simulink model "Target_Control_System"  (R2021b)
settings: Solver=FixedStepDiscrete  StartTime=0.0  StopTime=5  RelTol=1e-3
PreLoadFcn:
  | RTWConfigurationCB('preloadfcn', bdroot);
PostLoadFcn:
  | load('configuration/data_struct.mat');
  | load('configuration/fluxMaps_propMotor.mat');
  | load('configuration/parameterInit_PROP.mat');
  | load('configuration/parameterInit_PUMP.mat');
  | load('configuration/parameterInit_PITCH.mat');
  | load('configuration/parameterInit_TILT.mat');
  | %load('configuration/base_workspace_signal_definition.mat');
  | %load('resolvedatastores_to_baseworkspace_for_faster_simulation.mat');
model workspace (MAT data in the model file):
  SIMULATION_OPTIONS = Simulink.Parameter
  SIMULATION_OPTIONS.Value = 0
  SIMULATION_OPTIONS.Description = 'Set to ''0'' for normal Simulation
    | Set to ''1'' for "Flying Start" simulation'
  SIMULATION_OPTIONS.DataType = 'uint32'
  SIMULATION_OPTIONS.Complexity = 'real'
  SIMULATION_OPTIONS.Dimensions = [1 1]
  TARGET_CODE_GEN = Simulink.Parameter
  TARGET_CODE_GEN.Value = 0
  TARGET_CODE_GEN.Description = 'Set to ''0'' for Plant Model or PIL Simulation
    | Set to ''1'' for Target System Code Generation'
  TARGET_CODE_GEN.DataType = 'uint32'
  TARGET_CODE_GEN.Complexity = 'real'
  TARGET_CODE_GEN.Dimensions = [1 1]
  TCS_SAMPLE_FREQ_HZ = Simulink.Parameter
  TCS_SAMPLE_FREQ_HZ.Value = 160000
  TCS_SAMPLE_FREQ_HZ.DataType = 'double'
  TCS_SAMPLE_FREQ_HZ.Complexity = 'real'
  TCS_SAMPLE_FREQ_HZ.Dimensions = [1 1]
undefined symbols (not defined in the file): A_DQ_REF_LPF_INIT__PITCH, A_DQ_REF_LPF_INIT__PROP, A_DQ_REF_LPF_INIT__PUMP, A_DQ_REF_LPF_INIT__TILT, A_OBSERVER_CONFIDENCE_INIT__PITCH, A_OBSERVER_CONFIDENCE_INIT__PROP, A_OBSERVER_CONFIDENCE_INIT__PUMP, A_OBSERVER_CONFIDENCE_INIT__TILT, ACTUATOR_MAX_ANGLE_TRIP__PITCH, ACTUATOR_MIN_ANGLE_TRIP__PITCH, ACTUATOR_POS_SENSOR_INV_DIRECTION__PITCH, ACTUATOR_POS_SENSOR_INV_DIRECTION__TILT, ACTUATOR_POS_SENSOR_OFFSET__PITCH, ACTUATOR_POS_SENSOR_OFFSET__TILT, ADC_scaler1_baseaddr_TILT, ADC_SCALER_FLOAT_TO_FIXPOINT_EXPANSION, ANGLE_ELEC_FROM_SENSOR_OFFSET_INIT__PITCH, ANGLE_ELEC_FROM_SENSOR_OFFSET_INIT__PROP, ANGLE_ELEC_FROM_SENSOR_OFFSET_INIT__PUMP, ANGLE_ELEC_FROM_SENSOR_OFFSET_INIT__TILT, AUTO_CLEAR_FAULTS_ENABLED__PITCH, AUTO_CLEAR_FAULTS_ENABLED__PROP, AUTO_CLEAR_FAULTS_ENABLED__PUMP, AUTO_CLEAR_FAULTS_ENABLED__TILT, AUTO_CLEAR_FAULTS_WAIT_TICKS__PITCH, AUTO_CLEAR_FAULTS_WAIT_TICKS__PROP, AUTO_CLEAR_FAULTS_WAIT_TICKS__PUMP, AUTO_CLEAR_FAULTS_WAIT_TICKS__TILT, AUTO_I_ZERO_IDLE_TICKS__PITCH, AUTO_I_ZERO_IDLE_TICKS__PROP, AUTO_I_ZERO_IDLE_TICKS__PUMP, AUTO_I_ZERO_IDLE_TICKS__TILT, AUTO_I_ZERO_OFFSET_IDC_THRESHOLD__PITCH, AUTO_I_ZERO_OFFSET_IDC_THRESHOLD__PROP, AUTO_I_ZERO_OFFSET_IDC_THRESHOLD__PUMP, AUTO_I_ZERO_OFFSET_IDC_THRESHOLD__TILT, AUTO_I_ZERO_OFFSET_IPH_THRESHOLD__PITCH, AUTO_I_ZERO_OFFSET_IPH_THRESHOLD__PROP, AUTO_I_ZERO_OFFSET_IPH_THRESHOLD__PUMP, AUTO_I_ZERO_OFFSET_IPH_THRESHOLD__TILT, AUTO_SENSORLESS_SWITCHOVER_DISABLE_OMEGA, AUTO_SENSORLESS_SWITCHOVER_ENABLE_OMEGA, AUTO_SENSORLESS_SWITCHOVER_MIN_CONFIDENCE, AUXILIARY_PROTECTION_UNIT_BASEADDR__TILT, blanking_max_error_omega_INIT_PITCH, blanking_max_error_omega_INIT_TILT, blanking_max_error_position_INIT_PITCH, blanking_max_error_position_INIT_TILT, BRUTE_START_I_Q_REF_RAMP_SPEED__PITCH, BRUTE_START_I_Q_REF_RAMP_SPEED__PROP, BRUTE_START_I_Q_REF_RAMP_SPEED__PUMP, BRUTE_START_I_Q_REF_RAMP_SPEED__TILT, CONTROL_LOOP_DT_INIT__PITCH, CONTROL_LOOP_DT_INIT__PROP, CONTROL_LOOP_DT_INIT__PUMP, CONTROL_LOOP_DT_INIT__TILT, CORRECTION_FILTER_SCALE__PITCH, CORRECTION_FILTER_SCALE__PROP, CORRECTION_FILTER_SCALE__PUMP, CORRECTION_FILTER_SCALE__TILT ... (+458)
libraries: simulink x178, Reusables_Lib x24
(part 1 of 47)
settings Model: ModifiedComment=Brad -- Sat Feb 01 15:53:39 2014 -- Version 1.11  Creator=Brad Landseadel  LastModifiedBy=jessica.colton
settings Model: ModifiedHistory=|
  | Brad -- Sat Feb 01 15:53:39 2014 -- Version 1.11
  | 
  | 
  | Brad -- Sat Feb 01 15:53:39 2014 -- Version 1.11
  | 
  | 
  | Brad -- Sat Feb 01 15:48:49 2014 -- Version 1.10
  | 
  | 
  | Brad -- Sat Feb 01 15:38:18 2014 -- Version 1.9
  | 
  | 
  | Brad -- Sat Feb 01 15:22:57 2014 -- Version 1.8
  | 
  | 
  | Brad -- Sat Feb 01 15:08:45 2014 -- Version 1.7
  | 
  | 
  | Brad -- Sat Feb 01 14:46:18 2014 -- Version 1.6
  | 
  | 
  | Brad -- Sat Feb 01 13:34:06 2014 -- Version 1.5
  | 
  | 
  | Brad -- Sat Feb 01 13:29:08 2014 -- Version 1.4
  | 
  | 
  | Brad -- Sat Feb 01 13:18:41 2014 -- Version 1.3
  | 
  | 
  | Brad -- Sat Feb 01 12:30:13 2014 -- Version 1.2
settings SolverCC: AlgebraicLoopSolver=TrustRegion  PositivePriorityOrder=on
settings DataIOCC: LimitDataPoints=on  SaveFormat=Array  SignalLoggingSaveFormat=ModelDataLogs  SaveOutput=off  SaveTime=off  ReturnWorkspaceOutputs=off
settings OptimizationCC: DefaultParameterBehavior=Inlined  GainParamInheritBuiltInType=on  UseFloatMulNetSlope=on  DefaultUnderspecifiedDataType=single  InlineInvariantSignals=on  StrengthReduction=on  PassReuseOutputArgsAs=Individual arguments  ExpressionDepthLimit=2147483647  ZeroExternalMemoryAtStartup=off  ZeroInternalMemoryAtStartup=off  NoFixptDivByZeroProtection=on  EfficientFloat2IntCast=on  MaxStackSize=2000  SimCompilerOptimization=on  AccelVerboseBuild=on  OptimizeBlockOrder=speed  UseRowMajorAlgorithm=on  OptimizationPriority=Speed  LabelGuidedReuse=on  MultiThreadedLoops=on  EfficientTunableParamExpr=on
settings DebuggingCC: ReadBeforeWriteMsg=DisableAll  WriteAfterReadMsg=DisableAll  MergeDetectMultiDrivingBlocksExec=none  SolverPrmCheckMsg=warning  MultiTaskDSMMsg=none  MultiTaskRateTransMsg=warning  ParameterTunabilityLossMsg=error  FixptConstUnderflowMsg=error  FixptConstOverflowMsg=error  BusObjectLabelMismatch=error  AssertControl=DisableAll  AllowSymbolicDim=off  StateNameClashWarn=warning  SFUnexpectedBacktrackingDiag=warning  SFNoUnconditionalDefaultTransitionDiag=warning  SFExecutionAtInitializationDiag=none  SFMachineParentedDataDiag=warning  ArithmeticOperatorsInVariantConditions=warning
settings HardwareCC: ProdBitPerPointer=32  ProdBitPerSizeT=32  ProdBitPerPtrDiffT=32  ProdLargestAtomicInteger=Long  ProdLargestAtomicFloat=Double  ProdWordSize=32  ProdHWDeviceType=ARM Compatible->ARM Cortex-A  TargetLargestAtomicInteger=Long  TargetLargestAtomicFloat=Double  TargetIntDivRoundTo=Zero  TargetEndianess=LittleEndian  TargetHWDeviceType=ARM Compatible->ARM Cortex-A
settings ModelReferenceCC: UpdateModelReferenceTargets=IfOutOfDate  PropagateSignalLabelsOutOfModel=off
settings SFSimCC: SimCustomHeaderCode="//#include \"custom_code/second_level_include/math_special.h\""  SimUserSources=//math_special.c  SimUserIncludeDirs=//custom_code/src/  SFSimEcho=off  SimUseLocalCustomCode=off  MATLABDynamicMemAlloc=off  CustomCodeUndefinedFunction=UseInterfaceOnly
settings RTWCC: Description=Embedded Coder  SystemTargetFile=ert.tlc  GenCodeOnly=on  PackageGeneratedCodeAndArtifacts=on  TemplateMakefile=ert_default_tmf  GenerateReport=on  RetainRTWFile=on  RTWUseLocalCustomCode=off  CustomSource=custom_code/src/math_special.c  Toolchain=GNU gcc/g++ | gmake (64-bit Linux)  BuildConfiguration=Faster Runs  IncludeHyperlinkInReport=on  LaunchReport=on  GenerateTraceInfo=on  GenerateTraceReport=on  GenerateTraceReportSl=on  GenerateTraceReportSf=on  GenerateTraceReportEml=on  GenerateWebview=on  GenerateCodeMetricsReport=on  GenerateCodeReplacementReport=on  CheckMdlBeforeBuild=Warning
settings RTWCC: CustomHeaderCode=|
  | #include "../custom_code/second_level_include/math_special.h"
  | 
  | // FPGA interface
  | #include "../custom_code/include/motorTask_int.h"
  | #include "../custom_code/include/motorControl_common.h"
  | #include "../custom_code/include/common.h"
  | #include "../custom_code/include/motorControl_adc.h"
  | #include "../custom_code/include/motorControl_pwm.h"
  | 
  | // InterCore
  | #include "../custom_code/inverter_shared_memory/legacy_inverter_shared_memory_declaration.h"
  | 
  | // Second Level Includes
  | #include "../custom_code/second_level_include/adc.h"
  | #include "../custom_code/second_level_include/application_layer_com.h"
  | #include "../custom_code/second_level_include/gate_enable.h"
  | #include "../custom_code/second_level_include/housekeeping.h"
  | #include "../custom_code/second_level_include/hw_defines.h"
  | #include "../custom_code/second_level_include/iir.h"
  | #include "../custom_code/second_level_include/legacy_interCoreCom.h"
  | #include "../custom_code/second_level_include/motor_control_main.h"
  | #include "../custom_code/second_level_include/motorControl_common.h"
  | #include "../custom_code/second_level_include/motorTask_init.h"
  | #include "../custom_code/second_level_include/motorTask_intercoreCom.h"
  | #include "../custom_code/second_level_include/motorTask_main.h"
  | #include "../custom_code/second_level_include/motorTask_StateMachine.h"
  | #include "../custom_code/second_level_include/parameter_init.h"
  | #include "../custom_code/second_level_include/pattern_generator.h"
  | #include "../custom_code/second_level_include/pi_controller.h"
  | #include "../custom_code/second_level_include/platform.h"
  | #include "../custom_code/second_level_include/pwm.h"
  | #include "../custom_code/second_level_include/resolver_driver.h"
  | #include "../custom_code/second_level_include/software_identity_data_storage.h"
  | #include "../custom_code/second_level_include/std_math.h"
settings CodeAppCC: ForceParamTrailComments=on  IgnoreCustomStorageClasses=off  IgnoreTestpoints=on  MaxIdLength=128  OperatorAnnotations=on  SimulinkDataObjDesc=on  SFDataObjDesc=on  InsertBlockDesc=on  StateflowObjectComments=on
settings ERTTargetCC: TargetLangStandard=C99 (ISO)  CombineSignalStateStructs=on  GroupInternalDataByFunction=on  SuppressErrorStatus=on  SupportComplex=off  ParenthesesLevel=Maximum  CastingMode=Explicit  RootIOFormat=Structure reference  ERTCustomFileTemplate=example_file_process.tlc
settings ConfigComp: CovMetricSettings=dw  CovSaveCumulativeToWorkspaceVar=on  CovSaveSingleToWorkspaceVar=on  CovExternalEMLEnable=off  CovSFcnEnable=off
settings SimscapeCC: SimscapeNormalizeSystem=off

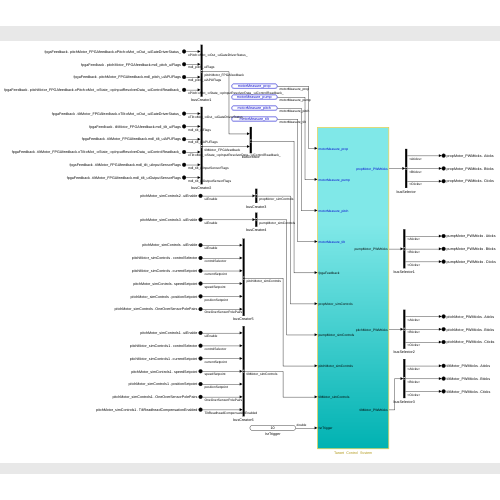
[thumbnail: Simulink's stored preview of the top-level diagram]
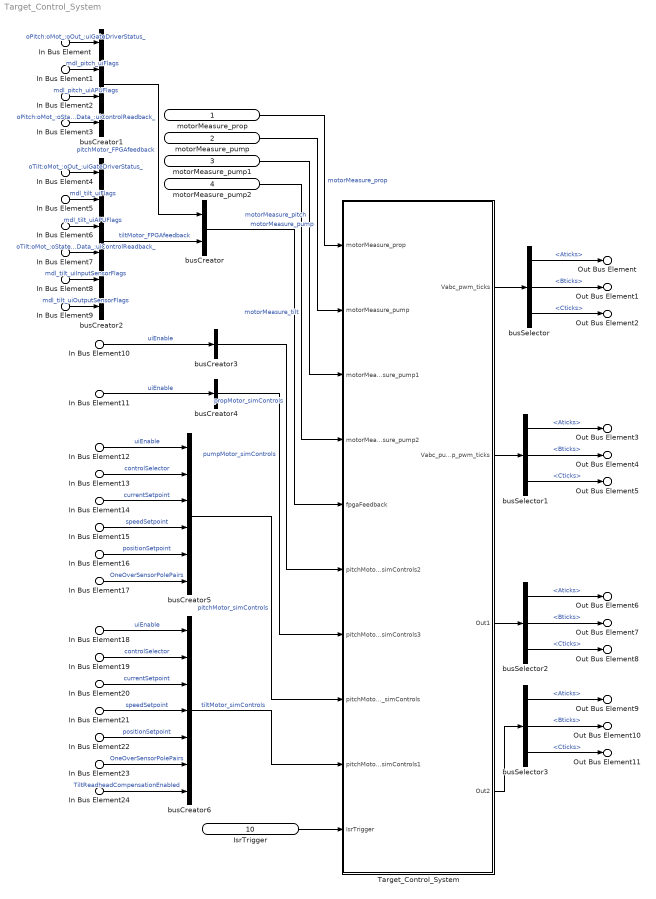
== system Target_Control_System ==
  motorMeasure_prop : Inport  OutDataTypeStr=Bus: SAdcDataSingleIn_t  SampleTime=[1/TCS_SAMPLE_FREQ_HZ,0]
  motorMeasure_pump : Inport  Port=2  OutDataTypeStr=Bus: SAdcDataSingleIn_t  SampleTime=[1/TCS_SAMPLE_FREQ_HZ,0]
  motorMeasure_pump1 : Inport  Port=3  OutDataTypeStr=Bus: SAdcDataSingleIn_t  SampleTime=[1/TCS_SAMPLE_FREQ_HZ,0]
  motorMeasure_pump2 : Inport  Port=4  OutDataTypeStr=Bus: SAdcDataSingleIn_t  SampleTime=[1/TCS_SAMPLE_FREQ_HZ,0]
  In Bus Element : Inport  Port=5  PortName=fpgaFeedback  Element=pitchMotor_FPGAfeedback.oPitch:oMot_:oOut_:uiGateDriverStatus_
  In Bus Element1 : Inport  Port=5  PortName=fpgaFeedback  Element=pitchMotor_FPGAfeedback.mdl_pitch_uiFlags
  In Bus Element2 : Inport  Port=5  PortName=fpgaFeedback  Element=pitchMotor_FPGAfeedback.mdl_pitch_uiAPUFlags
  In Bus Element3 : Inport  Port=5  PortName=fpgaFeedback  Element=pitchMotor_FPGAfeedback.oPitch:oMot_:oState_:opInputResolverData_:uiControlReadback_
  In Bus Element4 : Inport  Port=5  PortName=fpgaFeedback  Element=tiltMotor_FPGAfeedback.oTilt:oMot_:oOut_:uiGateDriverStatus_
  In Bus Element5 : Inport  Port=5  PortName=fpgaFeedback  Element=tiltMotor_FPGAfeedback.mdl_tilt_uiFlags
  In Bus Element6 : Inport  Port=5  PortName=fpgaFeedback  Element=tiltMotor_FPGAfeedback.mdl_tilt_uiAPUFlags
  In Bus Element7 : Inport  Port=5  PortName=fpgaFeedback  Element=tiltMotor_FPGAfeedback.oTilt:oMot_:oState_:opInputResolverData_:uiControlReadback_
  In Bus Element8 : Inport  Port=5  PortName=fpgaFeedback  Element=tiltMotor_FPGAfeedback.mdl_tilt_uiInputSensorFlags
  In Bus Element9 : Inport  Port=5  PortName=fpgaFeedback  Element=tiltMotor_FPGAfeedback.mdl_tilt_uiOutputSensorFlags
  In Bus Element10 : Inport  Port=6  PortName=pitchMotor_simControls2  Element=uiEnable
  In Bus Element11 : Inport  Port=7  PortName=pitchMotor_simControls3  Element=uiEnable
  In Bus Element12 : Inport  Port=8  PortName=pitchMotor_simControls  Element=uiEnable
  In Bus Element13 : Inport  Port=8  PortName=pitchMotor_simControls  Element=controlSelector
  In Bus Element14 : Inport  Port=8  PortName=pitchMotor_simControls  Element=currentSetpoint
  In Bus Element15 : Inport  Port=8  PortName=pitchMotor_simControls  Element=speedSetpoint
  In Bus Element16 : Inport  Port=8  PortName=pitchMotor_simControls  Element=positionSetpoint
  In Bus Element17 : Inport  Port=8  PortName=pitchMotor_simControls  Element=OneOverSensorPolePairs
  In Bus Element18 : Inport  Port=9  PortName=pitchMotor_simControls1  Element=uiEnable
  In Bus Element19 : Inport  Port=9  PortName=pitchMotor_simControls1  Element=controlSelector
  In Bus Element20 : Inport  Port=9  PortName=pitchMotor_simControls1  Element=currentSetpoint
  In Bus Element21 : Inport  Port=9  PortName=pitchMotor_simControls1  Element=speedSetpoint
  In Bus Element22 : Inport  Port=9  PortName=pitchMotor_simControls1  Element=positionSetpoint
  In Bus Element23 : Inport  Port=9  PortName=pitchMotor_simControls1  Element=OneOverSensorPolePairs
  In Bus Element24 : Inport  Port=9  PortName=pitchMotor_simControls1  Element=TiltReadheadCompensationEnabled
  IsrTrigger : Inport  Port=10  OutDataTypeStr=double  PortDimensions=1  SampleTime=1/TCS_SAMPLE_FREQ_HZ
  Target_Control_System : Subsystem  TreatAsAtomicUnit=on
  busCreator : BusCreator  Inputs=2
  busCreator1 : BusCreator  Inputs=4
  busCreator2 : BusCreator  Inputs=6
  busCreator3 : BusCreator  Inputs=1
  busCreator4 : BusCreator  Inputs=1
  busCreator5 : BusCreator  Inputs=6
  busCreator6 : BusCreator  Inputs=7
  busSelector{,1..3} (4 alike) : BusSelector  OutputSignals=Aticks,Bticks,Cticks
  Out Bus Element : Outport  PortName=propMotor_PWMticks  Element=Aticks
  Out Bus Element1 : Outport  PortName=propMotor_PWMticks  Element=Bticks
  Out Bus Element2 : Outport  PortName=propMotor_PWMticks  Element=Cticks
  Out Bus Element3 : Outport  Port=2  PortName=pumpMotor_PWMticks  Element=Aticks
  Out Bus Element4 : Outport  Port=2  PortName=pumpMotor_PWMticks  Element=Bticks
  Out Bus Element5 : Outport  Port=2  PortName=pumpMotor_PWMticks  Element=Cticks
  Out Bus Element6 : Outport  Port=3  PortName=pitchMotor_PWMticks  Element=Aticks
  Out Bus Element7 : Outport  Port=3  PortName=pitchMotor_PWMticks  Element=Bticks
  Out Bus Element8 : Outport  Port=3  PortName=pitchMotor_PWMticks  Element=Cticks
  Out Bus Element9 : Outport  Port=4  PortName=tiltMotor_PWMticks  Element=Aticks
  Out Bus Element10 : Outport  Port=4  PortName=tiltMotor_PWMticks  Element=Bticks
  Out Bus Element11 : Outport  Port=4  PortName=tiltMotor_PWMticks  Element=Cticks
  wires:
  motorMeasure_pump1/1 -> Target_Control_System/3(motorMeasure_pump1)  "motorMeasure_pitch"
  busCreator/1 -> Target_Control_System/5(fpgaFeedback)
  busCreator1/1 -> busCreator/1  "pitchMotor_FPGAfeedback"
  In Bus Element/1 -> busCreator1/1  "oPitch:oMot_:oOut_:uiGateDriverStatus_"
  In Bus Element2/1 -> busCreator1/3  "mdl_pitch_uiAPUFlags"
  In Bus Element4/1 -> busCreator2/1  "oTilt:oMot_:oOut_:uiGateDriverStatus_"
  In Bus Element1/1 -> busCreator1/2  "mdl_pitch_uiFlags"
  In Bus Element5/1 -> busCreator2/2  "mdl_tilt_uiFlags"
  In Bus Element7/1 -> busCreator2/4  "oTilt:oMot_:oState_:opInputResolverData_:uiControlReadback_"
  In Bus Element9/1 -> busCreator2/6  "mdl_tilt_uiOutputSensorFlags"
  busSelector/2 -> Out Bus Element1/1  "<Bticks>"
  busSelector3/3 -> Out Bus Element11/1  "<Cticks>"
  In Bus Element11/1 -> busCreator4/1  "uiEnable"
  busSelector2/3 -> Out Bus Element8/1  "<Cticks>"
  In Bus Element3/1 -> busCreator1/4  "oPitch:oMot_:oState_:opInputResolverData_:uiControlReadback_"
  busSelector1/1 -> Out Bus Element3/1  "<Aticks>"
  busSelector1/3 -> Out Bus Element5/1  "<Cticks>"
  In Bus Element23/1 -> busCreator6/6  "OneOverSensorPolePairs"
  Target_Control_System/2(Vabc_pump_pwm_ticks) -> busSelector1/1
  Target_Control_System/3(Out1) -> busSelector2/1
  motorMeasure_prop/1 -> Target_Control_System/1(motorMeasure_prop)  "motorMeasure_prop"
  busSelector3/2 -> Out Bus Element10/1  "<Bticks>"
  busSelector2/2 -> Out Bus Element7/1  "<Bticks>"
  Target_Control_System/4(Out2) -> busSelector3/1
  In Bus Element18/1 -> busCreator6/1  "uiEnable"
  busSelector1/2 -> Out Bus Element4/1  "<Bticks>"
  busSelector2/1 -> Out Bus Element6/1  "<Aticks>"
  In Bus Element8/1 -> busCreator2/5  "mdl_tilt_uiInputSensorFlags"
  busSelector3/1 -> Out Bus Element9/1  "<Aticks>"
  motorMeasure_pump2/1 -> Target_Control_System/4(motorMeasure_pump2)  "motorMeasure_tilt"
  In Bus Element6/1 -> busCreator2/3  "mdl_tilt_uiAPUFlags"
  In Bus Element24/1 -> busCreator6/7  "TiltReadheadCompensationEnabled"
  In Bus Element14/1 -> busCreator5/3  "currentSetpoint"
  Target_Control_System/1(Vabc_pwm_ticks) -> busSelector/1
  In Bus Element10/1 -> busCreator3/1  "uiEnable"
  In Bus Element12/1 -> busCreator5/1  "uiEnable"
  motorMeasure_pump/1 -> Target_Control_System/2(motorMeasure_pump)  "motorMeasure_pump"
  busCreator5/1 -> Target_Control_System/8(pitchMotor_simControls)  "pitchMotor_simControls"
  busSelector/1 -> Out Bus Element/1  "<Aticks>"
  In Bus Element22/1 -> busCreator6/5  "positionSetpoint"
  In Bus Element20/1 -> busCreator6/3  "currentSetpoint"
  In Bus Element21/1 -> busCreator6/4  "speedSetpoint"
  busCreator2/1 -> busCreator/2  "tiltMotor_FPGAfeedback"
  In Bus Element19/1 -> busCreator6/2  "controlSelector"
  In Bus Element17/1 -> busCreator5/6  "OneOverSensorPolePairs"
  In Bus Element16/1 -> busCreator5/5  "positionSetpoint"
  In Bus Element15/1 -> busCreator5/4  "speedSetpoint"
  busSelector/3 -> Out Bus Element2/1  "<Cticks>"
  In Bus Element13/1 -> busCreator5/2  "controlSelector"
  busCreator6/1 -> Target_Control_System/9(pitchMotor_simControls1)  "tiltMotor_simControls"
  busCreator4/1 -> Target_Control_System/7(pitchMotor_simControls3)  "pumpMotor_simControls"
  busCreator3/1 -> Target_Control_System/6(pitchMotor_simControls2)  "propMotor_simControls"
  IsrTrigger/1 -> Target_Control_System/10(IsrTrigger)

== system Target_Control_System/Target_Control_System ==
  motorMeasure_prop : Inport  OutDataTypeStr=Bus: SAdcDataSingleIn_t
  motorMeasure_pump : Inport  Port=2  OutDataTypeStr=Bus: SAdcDataSingleIn_t
  motorMeasure_pump1 : Inport  Port=3  OutDataTypeStr=Bus: SAdcDataSingleIn_t
  motorMeasure_pump2 : Inport  Port=4  OutDataTypeStr=Bus: SAdcDataSingleIn_t
  fpgaFeedback : Inport  Port=5
  pitchMotor_simControls2 : Inport  Port=6
  pitchMotor_simControls3 : Inport  Port=7
  pitchMotor_simControls : Inport  Port=8
  pitchMotor_simControls1 : Inport  Port=9
  IsrTrigger : Inport  Port=10
  Bus Creator2 : BusCreator  Inputs=4
  Constant1 : Constant  Value=TARGET_CODE_GEN == 0  OutDataTypeStr=boolean  SampleTime=-1
  Constant10 : Constant  Value=TARGET_CODE_GEN == 0  OutDataTypeStr=boolean  SampleTime=-1
  DEBUG_Scopes : Subsystem  TreatAsAtomicUnit=on  SystemSampleTime=1/((PWM_FREQ_KHZ__PROP*1000))*0.5
  Data Store Memory116 : DataStoreMemory  DataStoreName=fpga_uiPWMInterruptCount_  ReadBeforeWriteMsg=warning  WriteAfterWriteMsg=warning  WriteAfterReadMsg=warning  ShowAdditionalParam=off  OutDataTypeStr=uint32
  Data Store Memory16 : DataStoreMemory  DataStoreName=mdl_tilt_uiOutputSensorFlags  ReadBeforeWriteMsg=warning  WriteAfterWriteMsg=warning  WriteAfterReadMsg=warning  ShowAdditionalParam=off  OutDataTypeStr=uint32
  Data Store Memory19 : DataStoreMemory  DataStoreName=mdl_prop_fOmegaE  ReadBeforeWriteMsg=warning  WriteAfterWriteMsg=warning  WriteAfterReadMsg=warning  ShowAdditionalParam=off  OutDataTypeStr=single
  Data Store Memory2 : DataStoreMemory  DataStoreName=iCrossTripPitchToPropulsionMode  ReadBeforeWriteMsg=warning  WriteAfterWriteMsg=warning  WriteAfterReadMsg=warning  ShowAdditionalParam=off  OutDataTypeStr=uint32
  Data Store Memory29 : DataStoreMemory  DataStoreName=mdl_tilt_fOmegaE  ReadBeforeWriteMsg=warning  WriteAfterWriteMsg=warning  WriteAfterReadMsg=warning  ShowAdditionalParam=off  OutDataTypeStr=single
  Data Store Memory3 : DataStoreMemory  DataStoreName=mdl_pump_fOmegaE  ReadBeforeWriteMsg=warning  WriteAfterWriteMsg=warning  WriteAfterReadMsg=warning  ShowAdditionalParam=off  OutDataTypeStr=single
  Data Store Memory35 : DataStoreMemory  DataStoreName=mdl_tilt_uiFlags  ReadBeforeWriteMsg=warning  WriteAfterWriteMsg=warning  WriteAfterReadMsg=warning  ShowAdditionalParam=off  OutDataTypeStr=uint32
  Data Store Memory4 : DataStoreMemory  DataStoreName=mdl_pitch_uiInputSensorFlags  ReadBeforeWriteMsg=warning  WriteAfterWriteMsg=warning  WriteAfterReadMsg=warning  ShowAdditionalParam=off  OutDataTypeStr=uint32
  Data Store Memory42 : DataStoreMemory  DataStoreName=mdl_tilt_uiAPUFlags  ReadBeforeWriteMsg=warning  WriteAfterWriteMsg=warning  WriteAfterReadMsg=warning  ShowAdditionalParam=off  OutDataTypeStr=uint32
  Data Store Memory45 : DataStoreMemory  DataStoreName=mdl_pitch_fOmegaE  ReadBeforeWriteMsg=warning  WriteAfterWriteMsg=warning  WriteAfterReadMsg=warning  ShowAdditionalParam=off  OutDataTypeStr=single
  Data Store Memory5 : DataStoreMemory  DataStoreName=mdl_pitch_uiOutputSensorFlags  ReadBeforeWriteMsg=warning  WriteAfterWriteMsg=warning  WriteAfterReadMsg=warning  ShowAdditionalParam=off  OutDataTypeStr=uint32
  Data Store Memory51 : DataStoreMemory  DataStoreName=iCrossTripTiltToPropulsionMode  ReadBeforeWriteMsg=warning  WriteAfterWriteMsg=warning  WriteAfterReadMsg=warning  ShowAdditionalParam=off  OutDataTypeStr=uint32
  Data Store Memory6 : DataStoreMemory  DataStoreName=mdl_pitch_uiFlags  ReadBeforeWriteMsg=warning  WriteAfterWriteMsg=warning  WriteAfterReadMsg=warning  ShowAdditionalParam=off  OutDataTypeStr=uint32
  Data Store Memory7 : DataStoreMemory  DataStoreName=mdl_pitch_uiAPUFlags  ReadBeforeWriteMsg=warning  WriteAfterWriteMsg=warning  WriteAfterReadMsg=warning  ShowAdditionalParam=off  OutDataTypeStr=uint32
  Data Store Memory8 : DataStoreMemory  DataStoreName=fTemp  ReadBeforeWriteMsg=warning  WriteAfterWriteMsg=warning  WriteAfterReadMsg=warning  ShowAdditionalParam=off  OutDataTypeStr=single
  Data Store Memory9 : DataStoreMemory  DataStoreName=mdl_tilt_uiInputSensorFlags  ReadBeforeWriteMsg=warning  WriteAfterWriteMsg=warning  WriteAfterReadMsg=warning  ShowAdditionalParam=off  OutDataTypeStr=uint32
  Data Store Memory95 : DataStoreMemory  DataStoreName=oProp  ReadBeforeWriteMsg=warning  WriteAfterWriteMsg=warning  WriteAfterReadMsg=warning  ShowAdditionalParam=off  OutDataTypeStr=Bus: SMotorData_t
  Data Store Memory96 : DataStoreMemory  DataStoreName=oTilt  ReadBeforeWriteMsg=warning  WriteAfterWriteMsg=warning  WriteAfterReadMsg=warning  ShowAdditionalParam=off  OutDataTypeStr=Bus: SMotorData_t
  Data Store Memory97 : DataStoreMemory  DataStoreName=oPitch  ReadBeforeWriteMsg=warning  WriteAfterWriteMsg=warning  WriteAfterReadMsg=warning  ShowAdditionalParam=off  OutDataTypeStr=Bus: SMotorData_t
  Data Store Memory98 : DataStoreMemory  DataStoreName=oPump  ReadBeforeWriteMsg=warning  WriteAfterWriteMsg=warning  WriteAfterReadMsg=warning  ShowAdditionalParam=off  OutDataTypeStr=Bus: SMotorData_t
  DocBlock : simulink/Model-Wide Utilities/DocBlock  DocumentType=Text
      content=|
      | Setting up CCS v5.x for source code debugging with MATLAB generated source code
      |
      | 1) In the Code Generation Options under the Code Generation selection, click on the IDE Link option.
      | 2) Ensure that the Compiler option string: field includes  -g -D"_DEBUG"
      | 3) Generate code from within MATLAB
      |
      | Setting up CCS v5.x -- First time
      |
      | 1) Create or use a sample project within CCS to compile and connect to the target hardware. I used a simple PWM Trip Zone example.
      | 2) The debug perspective should open and you should now be connected to your hardware with the source code for the example open in the debug window.
      | 3) Close the code debug window for your example code. Do NOT terminate the debug session or disconnect from your hardware.
      | 4) Using the perspective tool buttons on the upper right of the toolbar in CCS, select the Edit perspective to go back to that perspective without disconnecting from your hardware.
      | 5) Once in the Edit perspective, create a new CCS project and define the appropriate processor and the same debug connection that was used in the example program to connect to the hardware.
      | 6) Once a new CCS project has been created, select that project in the project hierarchy pane to ensure it is open and selected.
      | 7) From the file menu, select Import and import the location of the MATLAB generated source files using the "File System" import method.
      | 8) Return to the Debug perspective using the toolbar on the top right of CCS v5.x.
      | 9) From the Run menu, select the Load option and navigate to the location--in the same path that you imported the file system above--of the .out file that was generated by the compiler and linker when you generated code from MATLAB.
      | Usually, this can be found in the DebugMW if you used the "Debug" configuration in the IDE Link dialog within MATLAB or from the CustomMW directory if you used a "Custom" configuration in the IDE Link dialog. Load this file.
      |
      | Code Composer Studio should have opened the "main" program in the source code window. You may now execute the code. Every time you hit the pause button and the execution halts within another source file, that file should open
      | automatically within the CCS debug perspective source code window. Alternatively, you can go back to the Edit perspective and open as many source files as you wish. Do NOT terminate your debug session when you do this, however.
      |
      | Setting up CCS v5.x -- After the first time
      |
      | 1) After generating code from MATLAB, complete steps 1 through 4 in Setting up CCS v5.x -- First time.
      | 2) After completing steps 1 through 4, select the project you created in in step 5 in the project hierarchy pane.
      | 3) Complete steps 8 and 9.
  InterruptFunction : Subsystem  TreatAsAtomicUnit=on  RTWFcnName=MotorControl_ISR
      settings: RTWFcnNameOpts=User specified
  MainLoop : Subsystem
  Model Info : simulink/Model-Wide Utilities/Model Info  Frame=on  DisplayStringWithTags=|  HorizontalTextAlignment=Center  LeftAlignmentValue=0.5
      | Model Info
      | %<ModelVersion>
      | %<ModifiedDate>
      | %<ModelName>
      | %<LastModificationDate>
      | %<ModifiedBy>
  ModelSource : Subsystem  Variant=on
  Rate Transition{4..7} (4 alike) : RateTransition  Deterministic=off
  Simulation Controls : Subsystem  TreatAsAtomicUnit=on
  System Start : Subsystem  Priority=30  mask(System Start){ShowInLibBrowser=0}
      mask prompts: ShowInLibBrowser "Simulink:masks:CustCodeMaskParam1_MP"
      settings: CopyFcn=cccopyfcn(gcb)  OpenFcn=ccopenfcn('System Start Function')
      mask Help: eval('feval(''rtwprivate'',''rtwhelpview'',''rtw_sys_start_block'')');
      mask Display: disp('System\nStart');
  Vabc_pwm_ticks : Outport
  Vabc_pump_pwm_ticks : Outport  Port=2
  Out1 : Outport  Port=3
  Out2 : Outport  Port=4
  wires:
  IsrTrigger/1 -> InterruptFunction/Trigger
  Rate Transition7/1 -> InterruptFunction/1(PropMotorAdcFeedback)
  Rate Transition4/1 -> InterruptFunction/2(PumpMotorAdcFeedback)
  Rate Transition5/1 -> InterruptFunction/3(PitchMotorAdcFeedback)
  Rate Transition6/1 -> InterruptFunction/4(TiltMotorAdcFeedback)
  MainLoop/4(Out4) -> Out2/1  "tiltMotor_PWMticks"
  MainLoop/3(Out3) -> [pitchMotor_PWMticks], Out1/1  "pitchMotor_PWMticks"
  MainLoop/2(Vabc_pump_pwm_ticks) -> Vabc_pump_pwm_ticks/1  "pumpMotor_PWMticks"
  MainLoop/1(Vabc_pwm_ticks) -> Vabc_pwm_ticks/1  "propMotor_PWMticks"
  fpgaFeedback/1 -> Simulation Controls/5(fpgaFeedback)  "fpgaFeedback"
  [pitchMotor_PWMticks] -> DEBUG_Scopes/2(pitchMotor_PWMticks)
  pitchMotor_simControls2/1 -> Simulation Controls/1(pitchMotor_simControls2)  "propMotor_simControls"
  pitchMotor_simControls3/1 -> Simulation Controls/2(pitchMotor_simControls3)  "pumpMotor_simControls"
  pitchMotor_simControls/1 -> Simulation Controls/3(pitchMotor_simControls)  "pitchMotor_simControls"
  pitchMotor_simControls1/1 -> Simulation Controls/4(pitchMotor_simControls1)  "tiltMotor_simControls"
  motorMeasure_prop/1 -> Rate Transition7/1, [motorFeedback_prop]  "motorMeasure_prop"
  motorMeasure_pump2/1 -> Rate Transition6/1, [motorFeedback_tilt]  "motorMeasure_tilt"
  motorMeasure_pump1/1 -> Rate Transition5/1, [motorFeedback_pitch]  "motorMeasure_pitch"
  motorMeasure_pump/1 -> Rate Transition4/1, [motorFeedback_pump]  "motorMeasure_pump"
  [motorFeedback_tilt] -> Bus Creator2/4
  [motorFeedback_prop] -> Bus Creator2/1
  Bus Creator2/1 -> DEBUG_Scopes/1(motorFeedback)  "motorFeedback"
  [motorFeedback_pitch] -> Bus Creator2/3
  [motorFeedback_pump] -> Bus Creator2/2
  Constant1/1 -> DEBUG_Scopes/Enable
  Constant10/1 -> Simulation Controls/Enable

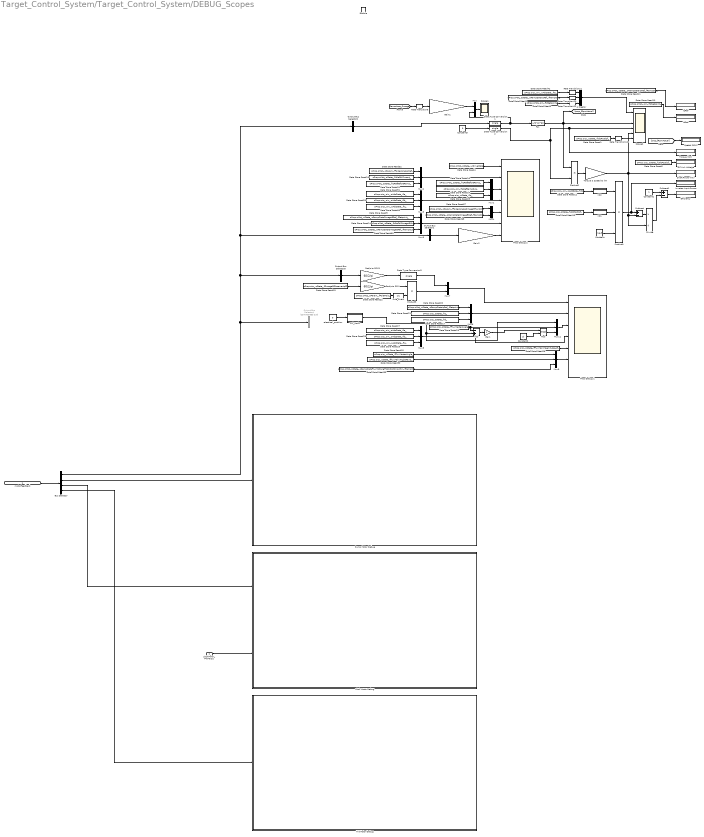
== system Target_Control_System/Target_Control_System/DEBUG_Scopes ==
  motorFeedback : Inport
  pitchMotor_PWMticks : Inport  Port=2
  Enable : EnablePort
  2Pi_Mod2 : Subsystem
  Add : Sum  Inputs=-+
  Bus Creator : BusCreator  Inputs=3
  Bus Selector : BusSelector  OutputSignals=motorMeasure_prop,motorMeasure_pump,motorMeasure_pitch,motorMeasure_tilt
  Constant : Constant  Value=1e-3  OutDataTypeStr=single  SampleTime=-1
  Constant1 : Constant  OutDataTypeStr=single  SampleTime=-1
  Constant2 : Constant  Value=pi  OutDataTypeStr=single  SampleTime=-1
  Constant3 : Constant  Value=0  OutDataTypeStr=single
  DC Link Voltage : Display
      settings: Format=decimal (Stored Integer)
  Data Store Read1 : DataStoreRead  DataStoreName=oProp  DataStoreElements=oProp.oIsr_.oState_.fUdcPostlpf_  IndexOptions=Index vector (dialog)  Indices=1  OutputSizes=1
  Data Store Read10 : DataStoreRead  DataStoreName=oProp  DataStoreElements=oProp.oMot_.oIn_.fIdSetpoint_  IndexOptions=Index vector (dialog)  Indices=1  OutputSizes=1
  Data Store Read11 : DataStoreRead  DataStoreName=oProp  DataStoreElements=oProp.oMot_.oState_.oRampDataIqRef_.fRampOut_  IndexOptions=Index vector (dialog)  Indices=1  OutputSizes=1
  Data Store Read12 : DataStoreRead  DataStoreName=oProp  DataStoreElements=oProp.oIsr_.oIn_.oAdcData_.fIdc_  IndexOptions=Index vector (dialog)  Indices=1  OutputSizes=1
  Data Store Read13 : DataStoreRead  DataStoreName=oProp  DataStoreElements=oProp.oIsr_.oState_.fUdcPostlpf_  IndexOptions=Index vector (dialog)  Indices=1  OutputSizes=1
  Data Store Read14 : DataStoreRead  DataStoreName=oProp  DataStoreElements=oProp.oMot_.oState_.fIdleCtrlOmegaEMin_  IndexOptions=Index vector (dialog)  Indices=1  OutputSizes=1
  Data Store Read15 : DataStoreRead  DataStoreName=oProp  DataStoreElements=oProp.oMot_.oState_.fIdleCtrlCurrent_  IndexOptions=Index vector (dialog)  Indices=1  OutputSizes=1
  Data Store Read16 : DataStoreRead  DataStoreName=oProp  DataStoreElements=oProp.oMot_.oState_.fIqRefBeforeRamp_  IndexOptions=Index vector (dialog)  Indices=1  OutputSizes=1
  Data Store Read17 : DataStoreRead  DataStoreName=oProp  DataStoreElements=oProp.oIsr_.oState_.fId_  IndexOptions=Index vector (dialog)  Indices=1  OutputSizes=1
  Data Store Read18 : DataStoreRead  DataStoreName=oProp  DataStoreElements=oProp.oIsr_.oState_.fFluxMasterAngle_  IndexOptions=Index vector (dialog)  Indices=1  OutputSizes=1
  Data Store Read19 : DataStoreRead  DataStoreName=oProp  DataStoreElements=oProp.oIsr_.oState_.fOmegaEObserverLpf2_  IndexOptions=Index vector (dialog)  Indices=1  OutputSizes=1
  Data Store Read2 : DataStoreRead  DataStoreName=oProp  DataStoreElements=oProp.oMot_.oState_.oRampDataIqRef_.fRampOut_  IndexOptions=Index vector (dialog)  Indices=1  OutputSizes=1
  Data Store Read20 : DataStoreRead  DataStoreName=oProp  DataStoreElements=oProp.oMot_.oState_.oRampDataIqRef_.fSetpoint_  IndexOptions=Index vector (dialog)  Indices=1  OutputSizes=1
  Data Store Read21 : DataStoreRead  DataStoreName=oProp  DataStoreElements=oProp.oIsr_.oState_.fIq_  IndexOptions=Index vector (dialog)  Indices=1  OutputSizes=1
  Data Store Read22 : DataStoreRead  DataStoreName=oProp  DataStoreElements=oProp.oMot_.oParam_.fPolePairs_  IndexOptions=Index vector (dialog)  Indices=1  OutputSizes=1
  Data Store Read23 : DataStoreRead  DataStoreName=oProp  DataStoreElements=oProp.oIsr_.oState_.fFluxMasterAngle_  IndexOptions=Index vector (dialog)  Indices=1  OutputSizes=1
  Data Store Read24 : DataStoreRead  DataStoreName=oProp  DataStoreElements=oProp.oIsr_.oIn_.fIqRefRampOut_  IndexOptions=Index vector (dialog)  Indices=1  OutputSizes=1
  Data Store Read25 : DataStoreRead  DataStoreName=oProp  DataStoreElements=oProp.oIsr_.oState_.fIq_  IndexOptions=Index vector (dialog)  Indices=1  OutputSizes=1
  Data Store Read26 : DataStoreRead  DataStoreName=oProp  DataStoreElements=oProp.oIsr_.oState_.fFluxMainMagnitudeLpf_  IndexOptions=Index vector (dialog)  Indices=1  OutputSizes=1
  Data Store Read27 : DataStoreRead  DataStoreName=oProp  DataStoreElements=oProp.oIsr_.oIn_.oAdcData_.fIa_  IndexOptions=Index vector (dialog)  Indices=1  OutputSizes=1
  Data Store Read28 : DataStoreRead  DataStoreName=oProp  DataStoreElements=oProp.oIsr_.oIn_.oAdcData_.fIb_  IndexOptions=Index vector (dialog)  Indices=1  OutputSizes=1
  Data Store Read29 : DataStoreRead  DataStoreName=oProp  DataStoreElements=oProp.oIsr_.oIn_.oAdcData_.fIc_  IndexOptions=Index vector (dialog)  Indices=1  OutputSizes=1
  Data Store Read30 : DataStoreRead  DataStoreName=oProp  DataStoreElements=oProp.oIsr_.oState_.fFluxMainAngleRaw2_  IndexOptions=Index vector (dialog)  Indices=1  OutputSizes=1
  Data Store Read31 : DataStoreRead  DataStoreName=oProp  DataStoreElements=oProp.oMot_.oState_.fIqRefBeforeRamp_  IndexOptions=Index vector (dialog)  Indices=1  OutputSizes=1
  Data Store Read32 : DataStoreRead  DataStoreName=oProp  DataStoreElements=oProp.oMot_.oParam_.fForcedAngleIRef_  IndexOptions=Index vector (dialog)  Indices=1  OutputSizes=1
  Data Store Read33 : DataStoreRead  DataStoreName=oProp  DataStoreElements=oProp.oMot_.oState_.oRampDataFluxMstrAngFrcd2clsdSmoothn_.fRampOut_  IndexOptions=Index vector (dialog)  Indices=1  OutputSizes=1
  Data Store Read4 : DataStoreRead  DataStoreName=oProp  DataStoreElements=oProp.oMot_.oState_.uiDriveState_  IndexOptions=Index vector (dialog)  Indices=1  OutputSizes=1
  Data Store Read42 : DataStoreRead  DataStoreName=oProp  DataStoreElements=oProp.oIsr_.oIn_.oAdcData_.fIa_  IndexOptions=Index vector (dialog)  Indices=1  OutputSizes=1
  Data Store Read5 : DataStoreRead  DataStoreName=oProp  DataStoreElements=oProp.oMot_.oIn_.fIdSetpoint_  IndexOptions=Index vector (dialog)  Indices=1  OutputSizes=1
  Data Store Read51 : DataStoreRead  DataStoreName=oProp  DataStoreElements=oProp.oIsr_.oIn_.oAdcData_.fIa_  IndexOptions=Index vector (dialog)  Indices=1  OutputSizes=1
  Data Store Read53 : DataStoreRead  DataStoreName=oProp  DataStoreElements=oProp.oIsr_.oIn_.oAdcData_.fIb_  IndexOptions=Index vector (dialog)  Indices=1  OutputSizes=1
  Data Store Read6 : DataStoreRead  DataStoreName=oProp  DataStoreElements=oProp.oIsr_.oState_.fUdcPostlpf_  IndexOptions=Index vector (dialog)  Indices=1  OutputSizes=1
  Data Store Read66 : DataStoreRead  DataStoreName=oProp  DataStoreElements=oProp.oIsr_.oIn_.oAdcData_.fIc_  IndexOptions=Index vector (dialog)  Indices=1  OutputSizes=1
  Data Store Read67 : DataStoreRead  DataStoreName=oProp  DataStoreElements=oProp.oMot_.oParam_.fForcedAngleOmegaEHandoff_  IndexOptions=Index vector (dialog)  Indices=1  OutputSizes=1
  Data Store Read68 : DataStoreRead  DataStoreName=oProp  DataStoreElements=oProp.oMot_.oState_.oRampDataOmegaERef_.fRampOut_  IndexOptions=Index vector (dialog)  Indices=1  OutputSizes=1
  Data Store Read69 : DataStoreRead  DataStoreName=oProp  DataStoreElements=oProp.oMot_.oState_.oRampDataOmegaERef_.fRampOut_  IndexOptions=Index vector (dialog)  Indices=1  OutputSizes=1
  Data Store Read9 : DataStoreRead  DataStoreName=oProp  DataStoreElements=oProp.oMot_.oState_.oRampDataOmegaERef_.fSetpoint_  IndexOptions=Index vector (dialog)  Indices=1  OutputSizes=1
  Data Type Conversion1 : DataTypeConversion  OutDataTypeStr=single
  Data Type Conversion2 : DataTypeConversion  OutDataTypeStr=single
  Data Type Conversion3 : DataTypeConversion  OutDataTypeStr=single
  Divide : Product  Inputs=*/
  Efficiency : Display
      settings: Format=decimal (Stored Integer)
  Fcn : Fcn  Expr=u/(2*pi)*60
  Gain : Gain
  Gain1 : Gain  Gain=1/POLE_PAIRS_INIT__PROP
  Gain2 : Gain  Gain=POLE_PAIRS_INIT__PROP
  IIR1 : Subsystem  mask{CoefficientA=0.7, CoefficientB=0.3}
      mask prompts: CoefficientA "First Coefficient (long)"; CoefficientB "Second Coefficient (short)"
  IIR2 : Subsystem  mask{CoefficientA=0.7, CoefficientB=0.3}
      mask prompts: CoefficientA "First Coefficient (long)"; CoefficientB "Second Coefficient (short)"
  IdRef : Display
      settings: Format=decimal (Stored Integer)
  Inverter Input Power : Display
      settings: Format=decimal (Stored Integer)
  IqRef : Display
      settings: Format=decimal (Stored Integer)
  Mod : Math  Operator=mod  SaturateOnIntegerOverflow=on
  Mux : Mux  Inputs=2
  Mux{1..3,5..6,8..9,11} (8 alike) : Mux  Inputs=3
  Mux4 : Mux  Inputs=2
  Mux7 : Mux  Inputs=2
  One_Over1 : Fcn  Expr=1/u
  Output Bus Selector1 : BusSelector  OutputSignals=fMotorSensorSpeed_
  Output Bus Selector2 : BusSelector  OutputSignals=fMotorSensorSpeed_
  Output Bus Selector3 : BusSelector  OutputSignals=fMotorSensorSpeed_
  Output Bus Selector4 : BusSelector  Commented=on  OutputSignals=position_electrical_prop
  Pitch Motor Debug : Subsystem
  Product1 : Product  Inputs=3
  Product2 : Product
  Product3 : Product
  Prop Debug 1 : Scope  NumInputPorts=7
  Prop Debug 2 : Scope  NumInputPorts=7
  Pump Motor Debug : Subsystem
  Rad/s to RPM : Gain  Gain=60/2/pi  OutDataTypeStr=single
  Rad/s to RPM1 : Gain  Gain=60/2/pi  OutDataTypeStr=single
  Rate Transition{6,10,20..22} (5 alike) : RateTransition  Deterministic=off
  Scope1 : Scope
  Scope2 : Scope  NumInputPorts=6
  Shaft Power (kW) : Display
      settings: Format=decimal (Stored Integer)
  Speed (RPM) : Display
      settings: Format=decimal (Stored Integer)
  Subtract : Sum  Inputs=+-
  Subtract1 : Sum  Inputs=+-
  Tilt Motor Debug : Subsystem
  Torque & Speed to kW : Gain  Gain=1/9.5488*1e-3
  Torque (Nm) : Display
      settings: Format=decimal (Stored Integer)
  electrical_position : Constant  Value=0  OutDataTypeStr=single
  wires:
  electrical_position/1 -> 2Pi_Mod2/1(Iabc1)
  pitchMotor_PWMticks/1 -> Pitch Motor Debug/2(pitchMotor_PWMticks)
  Bus Selector/4 -> Tilt Motor Debug/1(In1)  "<motorMeasure_tilt>"
  Mod/1 -> Mux11/3
  Gain/1 -> Mod/1
  Constant2/1 -> Mod/2
  2Pi_Mod2/1(Out1) -> Mux11/1, Add/2
  Bus Selector/2 -> Pump Motor Debug/1(In1)  "<motorMeasure_pump>"
  Bus Selector/3 -> Pitch Motor Debug/1(In1)  "<motorMeasure_pitch>"
  Bus Selector/1 -> Output Bus Selector3/1, Output Bus Selector1/1, Output Bus Selector2/1, Output Bus Selector4/1  "<motorMeasure_prop>"
  motorFeedback/1 -> Bus Selector/1
  Data Store Read33/1 -> Mux9/3
  Data Store Read23/1 -> Mux11/2, Add/1
  Mux6/1 -> Prop Debug 1/2
  Data Store Read21/1 -> Mux6/2
  Data Store Read17/1 -> Mux6/3
  Rad/s to RPM/1 -> Product3/1
  Output Bus Selector3/1 -> Rad/s to RPM1/1  "<fMotorSensorSpeed_>"
  Mux8/1 -> Prop Debug 1/4
  Product3/1 -> Mux7/2
  Mux9/1 -> Prop Debug 1/6
  Mux7/1 -> Prop Debug 1/1
  Data Store Read18/1 -> Mux9/1
  Data Store Read29/1 -> Mux8/3
  Data Store Read28/1 -> Mux8/2
  Data Store Read20/1 -> Mux6/1
  One_Over1/1 -> Product3/2
  Data Store Read27/1 -> Mux8/1
  Add/1 -> Gain/1
  Rad/s to RPM1/1 -> Data Type Conversion3/1
  Data Store Read30/1 -> Mux9/2
  Mux11/1 -> Prop Debug 1/3
  Data Store Read19/1 -> Rad/s to RPM/1
  Data Type Conversion3/1 -> Mux7/1
  Data Store Read22/1 -> One_Over1/1
  Data Store Read26/1 -> Prop Debug 1/5
  Gain2/1 -> Prop Debug 2/7
  Output Bus Selector1/1 -> Gain2/1  "<fMotorSensorSpeed_>"
  Data Store Read51/1 -> Mux3/1
  Data Store Read53/1 -> Mux3/2
  Data Store Read9/1 -> Mux5/1
  Mux1/1 -> Prop Debug 2/3
  Mux4/1 -> Prop Debug 2/5
  Data Store Read31/1 -> Mux2/3  "fIdleCtrlCurrent_"
  Data Store Read4/1 -> Prop Debug 2/1
  Mux3/1 -> Prop Debug 2/4
  Data Store Read67/1 -> Mux4/1
  Data Store Read15/1 -> Mux2/2
  Data Store Read69/1 -> Mux5/3
  Data Store Read14/1 -> Mux5/2
  Data Store Read24/1 -> Mux1/2
  Data Store Read68/1 -> Mux4/2
  Data Store Read66/1 -> Mux3/3
  Mux5/1 -> Prop Debug 2/6
  Data Store Read16/1 -> Mux1/1
  Mux2/1 -> Prop Debug 2/2
  Data Store Read25/1 -> Mux1/3
  Data Store Read32/1 -> Mux2/1
  Subtract/1 -> Divide/1
  Data Store Read2/1 -> Rate Transition20/1
  Data Store Read5/1 -> Rate Transition22/1
  IIR1/1(Output) -> Product1/2
  Data Store Read11/1 -> IqRef/1
  Constant3/1 -> Data Type Conversion2/1  "<torque_prop>"
  Product2/1 -> Torque & Speed to kW/1
  Output Bus Selector2/1 -> Data Type Conversion1/1  "<fMotorSensorSpeed_>"
  Data Store Read42/1 -> Rate Transition21/1
  Data Store Read1/1 -> Rate Transition10/1
  Rate Transition20/1 -> Bus Creator/2
  Data Store Read13/1 -> IIR1/1(Input)
  Data Store Read12/1 -> IIR2/1(Input)
  [Sensorless_Omega] -> Rate Transition6/1
  Mux/1 -> Scope1/1
  Rate Transition22/1 -> Bus Creator/3
  Rate Transition6/1 -> Gain1/1
  Data Type Conversion2/1 -> Product2/2, Scope2/4, Torque (Nm)/1
  Data Store Read10/1 -> IdRef/1
  Constant1/1 -> Subtract1/1
  Product1/1 -> Inverter Input Power/1, Subtract/1
  Bus Creator/1 -> Scope2/1
  Gain1/1 -> Mux/1
  Torque & Speed to kW/1 -> Scope2/5, Subtract/2, Divide/2, Shaft Power (kW)/1  "ShaftPower"
  Constant/1 -> Product1/3
  Fcn/1 -> Scope2/3, Product2/1, [prop_fRpmActual]
  Rate Transition10/1 -> Scope2/6
  Subtract1/1 -> Efficiency/1
  IIR2/1(Output) -> Product1/1
  Data Type Conversion1/1 -> Mux/2, Fcn/1
  Data Store Read6/1 -> DC Link Voltage/1
  Rate Transition21/1 -> Bus Creator/1
  Divide/1 -> Subtract1/2
  [prop_fRpmActual] -> Speed (RPM)/1

== system Target_Control_System/Target_Control_System/InterruptFunction ==
  In Bus Element : Inport  PortName=PropMotorAdcFeedback
  In Bus Element1 : Inport  Port=2  PortName=PumpMotorAdcFeedback
  In Bus Element2 : Inport  Port=3  PortName=PitchMotorAdcFeedback
  In Bus Element3 : Inport  Port=4  PortName=TiltMotorAdcFeedback
  Trigger : TriggerPort  VariantControl=(inherit)  PortDimensions=1
  Data Store Memory10 : DataStoreMemory  DataStoreName=mdl_pump_fUphFilterDelayAngleRad_cos_  ReadBeforeWriteMsg=warning  WriteAfterWriteMsg=warning  WriteAfterReadMsg=warning  ShowAdditionalParam=off  OutDataTypeStr=single
  Data Store Memory11 : DataStoreMemory  DataStoreName=mdl_pitch_fUphFilterDelayAngleRad_cos_  ReadBeforeWriteMsg=warning  WriteAfterWriteMsg=warning  WriteAfterReadMsg=warning  ShowAdditionalParam=off  OutDataTypeStr=single
  Data Store Memory12 : DataStoreMemory  DataStoreName=mdl_pump_fFluxMasterAngle_sin_  ReadBeforeWriteMsg=warning  WriteAfterWriteMsg=warning  WriteAfterReadMsg=warning  ShowAdditionalParam=off  OutDataTypeStr=single
  Data Store Memory13 : DataStoreMemory  DataStoreName=mdl_pitch_fFluxMasterAngle_sin_  ReadBeforeWriteMsg=warning  WriteAfterWriteMsg=warning  WriteAfterReadMsg=warning  ShowAdditionalParam=off  OutDataTypeStr=single
  Data Store Memory14 : DataStoreMemory  DataStoreName=mdl_pitch_fFluxMasterAngle_cos_  ReadBeforeWriteMsg=warning  WriteAfterWriteMsg=warning  WriteAfterReadMsg=warning  ShowAdditionalParam=off  OutDataTypeStr=single
  Data Store Memory15 : DataStoreMemory  DataStoreName=mdl_pitch_fFluxMainAngleRaw2_sin_  ReadBeforeWriteMsg=warning  WriteAfterWriteMsg=warning  WriteAfterReadMsg=warning  ShowAdditionalParam=off  OutDataTypeStr=single
  Data Store Memory17 : DataStoreMemory  DataStoreName=mdl_pitch_fFluxMainAngleRaw2_cos_  ReadBeforeWriteMsg=warning  WriteAfterWriteMsg=warning  WriteAfterReadMsg=warning  ShowAdditionalParam=off  OutDataTypeStr=single
  Data Store Memory18 : DataStoreMemory  DataStoreName=mdl_pitch_fFluxMasterAngleBkwd_sin_  ReadBeforeWriteMsg=warning  WriteAfterWriteMsg=warning  WriteAfterReadMsg=warning  ShowAdditionalParam=off  OutDataTypeStr=single
  Data Store Memory20 : DataStoreMemory  DataStoreName=mdl_pitch_fFluxMasterAngleBkwd_cos_  ReadBeforeWriteMsg=warning  WriteAfterWriteMsg=warning  WriteAfterReadMsg=warning  ShowAdditionalParam=off  OutDataTypeStr=single
  Data Store Memory21 : DataStoreMemory  DataStoreName=mdl_pitch_fUphFilterDelayAngleRad_sin_  ReadBeforeWriteMsg=warning  WriteAfterWriteMsg=warning  WriteAfterReadMsg=warning  ShowAdditionalParam=off  OutDataTypeStr=single
  Data Store Memory27 : DataStoreMemory  DataStoreName=mdl_tilt_fUphFilterDelayAngleRad_cos_  ReadBeforeWriteMsg=warning  WriteAfterWriteMsg=warning  WriteAfterReadMsg=warning  ShowAdditionalParam=off  OutDataTypeStr=single
  Data Store Memory30 : DataStoreMemory  DataStoreName=mdl_tilt_fFluxMasterAngle_sin_  ReadBeforeWriteMsg=warning  WriteAfterWriteMsg=warning  WriteAfterReadMsg=warning  ShowAdditionalParam=off  OutDataTypeStr=single
  Data Store Memory31 : DataStoreMemory  DataStoreName=mdl_tilt_fFluxMasterAngle_cos_  ReadBeforeWriteMsg=warning  WriteAfterWriteMsg=warning  WriteAfterReadMsg=warning  ShowAdditionalParam=off  OutDataTypeStr=single
  Data Store Memory32 : DataStoreMemory  DataStoreName=mdl_tilt_fFluxMainAngleRaw2_sin_  ReadBeforeWriteMsg=warning  WriteAfterWriteMsg=warning  WriteAfterReadMsg=warning  ShowAdditionalParam=off  OutDataTypeStr=single
  Data Store Memory36 : DataStoreMemory  DataStoreName=mdl_tilt_fFluxMainAngleRaw2_cos_  ReadBeforeWriteMsg=warning  WriteAfterWriteMsg=warning  WriteAfterReadMsg=warning  ShowAdditionalParam=off  OutDataTypeStr=single
  Data Store Memory37 : DataStoreMemory  DataStoreName=mdl_tilt_fFluxMasterAngleBkwd_sin_  ReadBeforeWriteMsg=warning  WriteAfterWriteMsg=warning  WriteAfterReadMsg=warning  ShowAdditionalParam=off  OutDataTypeStr=single
  Data Store Memory38 : DataStoreMemory  DataStoreName=mdl_tilt_fFluxMasterAngleBkwd_cos_  ReadBeforeWriteMsg=warning  WriteAfterWriteMsg=warning  WriteAfterReadMsg=warning  ShowAdditionalParam=off  OutDataTypeStr=single
  Data Store Memory39 : DataStoreMemory  DataStoreName=mdl_tilt_fUphFilterDelayAngleRad_sin_  ReadBeforeWriteMsg=warning  WriteAfterWriteMsg=warning  WriteAfterReadMsg=warning  ShowAdditionalParam=off  OutDataTypeStr=single
  Data Store Memory41 : DataStoreMemory  DataStoreName=mdl_pump_fFluxMasterAngle_cos_  ReadBeforeWriteMsg=warning  WriteAfterWriteMsg=warning  WriteAfterReadMsg=warning  ShowAdditionalParam=off  OutDataTypeStr=single
  Data Store Memory43 : DataStoreMemory  DataStoreName=mdl_fFluxMasterAngle_sin_  ReadBeforeWriteMsg=warning  WriteAfterWriteMsg=warning  WriteAfterReadMsg=warning  ShowAdditionalParam=off  OutDataTypeStr=single
  Data Store Memory44 : DataStoreMemory  DataStoreName=mdl_fFluxMasterAngle_cos_  ReadBeforeWriteMsg=warning  WriteAfterWriteMsg=warning  WriteAfterReadMsg=warning  ShowAdditionalParam=off  OutDataTypeStr=single
  Data Store Memory46 : DataStoreMemory  DataStoreName=mdl_fFluxMainAngleRaw2_sin_  ReadBeforeWriteMsg=warning  WriteAfterWriteMsg=warning  WriteAfterReadMsg=warning  ShowAdditionalParam=off  OutDataTypeStr=single
  Data Store Memory49 : DataStoreMemory  DataStoreName=mdl_fFluxMainAngleRaw2_cos_  ReadBeforeWriteMsg=warning  WriteAfterWriteMsg=warning  WriteAfterReadMsg=warning  ShowAdditionalParam=off  OutDataTypeStr=single
  Data Store Memory50 : DataStoreMemory  DataStoreName=mdl_fFluxMasterAngleBkwd_sin_  ReadBeforeWriteMsg=warning  WriteAfterWriteMsg=warning  WriteAfterReadMsg=warning  ShowAdditionalParam=off  OutDataTypeStr=single
  Data Store Memory52 : DataStoreMemory  DataStoreName=mdl_fFluxMasterAngleBkwd_cos_  ReadBeforeWriteMsg=warning  WriteAfterWriteMsg=warning  WriteAfterReadMsg=warning  ShowAdditionalParam=off  OutDataTypeStr=single
  Data Store Memory53 : DataStoreMemory  DataStoreName=mdl_pump_fFluxMainAngleRaw2_sin_  ReadBeforeWriteMsg=warning  WriteAfterWriteMsg=warning  WriteAfterReadMsg=warning  ShowAdditionalParam=off  OutDataTypeStr=single
  Data Store Memory55 : DataStoreMemory  DataStoreName=mdl_pump_fFluxMainAngleRaw2_cos_  ReadBeforeWriteMsg=warning  WriteAfterWriteMsg=warning  WriteAfterReadMsg=warning  ShowAdditionalParam=off  OutDataTypeStr=single
  Data Store Memory56 : DataStoreMemory  DataStoreName=mdl_pump_fFluxMasterAngleBkwd_sin_  ReadBeforeWriteMsg=warning  WriteAfterWriteMsg=warning  WriteAfterReadMsg=warning  ShowAdditionalParam=off  OutDataTypeStr=single
  Data Store Memory57 : DataStoreMemory  DataStoreName=mdl_pump_fFluxMasterAngleBkwd_cos_  ReadBeforeWriteMsg=warning  WriteAfterWriteMsg=warning  WriteAfterReadMsg=warning  ShowAdditionalParam=off  OutDataTypeStr=single
  Data Store Memory58 : DataStoreMemory  DataStoreName=mdl_fUphFilterDelayAngleRad_sin_  ReadBeforeWriteMsg=warning  WriteAfterWriteMsg=warning  WriteAfterReadMsg=warning  ShowAdditionalParam=off  OutDataTypeStr=single
  Data Store Memory59 : DataStoreMemory  DataStoreName=mdl_fUphFilterDelayAngleRad_cos_  ReadBeforeWriteMsg=warning  WriteAfterWriteMsg=warning  WriteAfterReadMsg=warning  ShowAdditionalParam=off  OutDataTypeStr=single
  Data Store Memory60 : DataStoreMemory  DataStoreName=mdl_pump_fUphFilterDelayAngleRad_sin_  ReadBeforeWriteMsg=warning  WriteAfterWriteMsg=warning  WriteAfterReadMsg=warning  ShowAdditionalParam=off  OutDataTypeStr=single
  Data Store Memory62 : DataStoreMemory  DataStoreName=mdl_suiIsrSmallInvCounter_  ReadBeforeWriteMsg=warning  WriteAfterWriteMsg=warning  WriteAfterReadMsg=warning  ShowAdditionalParam=off  OutDataTypeStr=uint32
  Function-Call Generator : simulink/Ports & Subsystems/Function-Call Generator  sample_time=-1  numberOfIterations=1  DisallowWideOutput=off
  Function-Call Split{,1..15} (16 alike) : FunctionCallSplit  NumOutputPorts=2
  allMotors_readAdc : Subsystem  TreatAsAtomicUnit=on
  pitchMotor_dataToIsr : Subsystem  TreatAsAtomicUnit=on
  pitchMotor_dataToMain : Subsystem  TreatAsAtomicUnit=on
  pitchMotor_isrSchedule : Subsystem  TreatAsAtomicUnit=on
  pitchMotor_isrTask : Subsystem
  pitchMotor_setPwm : Subsystem  TreatAsAtomicUnit=on
  propMotor_IsrSchedule : Subsystem  TreatAsAtomicUnit=on
  propMotor_dataToIsr : Subsystem  TreatAsAtomicUnit=on
  propMotor_dataToMain : Subsystem  TreatAsAtomicUnit=on
  propMotor_isrTask : Subsystem
  propMotor_setPwm : Subsystem  TreatAsAtomicUnit=on
  pumpMotor_dataToIsr : Subsystem  TreatAsAtomicUnit=on
  pumpMotor_dataToMain : Subsystem  TreatAsAtomicUnit=on
  pumpMotor_isrSchedule : Subsystem  TreatAsAtomicUnit=on
  pumpMotor_isrTask : Subsystem
  pumpMotor_setPwm : Subsystem  TreatAsAtomicUnit=on
  tiltMotor_dataToIsr : Subsystem  TreatAsAtomicUnit=on
  tiltMotor_dataToMain : Subsystem  TreatAsAtomicUnit=on
  tiltMotor_isrSchedule : Subsystem  TreatAsAtomicUnit=on
  tiltMotor_isrTask : Subsystem
  tiltMotor_setPwm : Subsystem  TreatAsAtomicUnit=on
  wires:
  Function-Call Generator/1 -> propMotor_IsrSchedule/Trigger
  Function-Call Split11/2 -> Function-Call Split6/1
  Function-Call Split6/1 -> tiltMotor_isrTask/Trigger
  Function-Call Split13/1 -> pitchMotor_dataToIsr/Trigger
  Function-Call Split2/1 -> propMotor_isrTask/Trigger
  Function-Call Split/1 -> allMotors_readAdc/Trigger
  Function-Call Split3/2 -> Function-Call Split4/1
  Function-Call Split4/1 -> propMotor_dataToMain/Trigger
  In Bus Element2/1 -> allMotors_readAdc/3(PitchMotorAdcFeedback)
  Function-Call Split5/2 -> pitchMotor_isrSchedule/Trigger
  Function-Call Split1/2 -> Function-Call Split2/1
  In Bus Element3/1 -> allMotors_readAdc/4(TiltMotorAdcFeedback)
  Function-Call Split6/2 -> Function-Call Split12/1
  Function-Call Split12/2 -> tiltMotor_dataToMain/Trigger
  Function-Call Split/2 -> Function-Call Split1/1
  Function-Call Split14/1 -> pitchMotor_isrTask/Trigger
  Function-Call Split3/1 -> propMotor_setPwm/Trigger
  Function-Call Split4/2 -> Function-Call Split7/1
  Function-Call Split15/1 -> pitchMotor_setPwm/Trigger
  Function-Call Split9/2 -> Function-Call Split8/1
  In Bus Element1/1 -> allMotors_readAdc/2(PumpMotorAdcFeedback)
  Function-Call Split10/1 -> pumpMotor_setPwm/Trigger
  Function-Call Split2/2 -> Function-Call Split3/1
  Function-Call Split13/2 -> Function-Call Split14/1
  Function-Call Split15/2 -> pitchMotor_dataToMain/Trigger
  Function-Call Split8/2 -> Function-Call Split10/1
  Function-Call Split12/1 -> tiltMotor_setPwm/Trigger
  propMotor_IsrSchedule/1(IsrEnable) -> Function-Call Split/1
  pitchMotor_isrSchedule/1(Output) -> Function-Call Split13/1
  Function-Call Split1/1 -> propMotor_dataToIsr/Trigger
  Function-Call Split10/2 -> pumpMotor_dataToMain/Trigger
  pumpMotor_isrSchedule/1(Output) -> Function-Call Split9/1
  Function-Call Split8/1 -> pumpMotor_isrTask/Trigger
  Function-Call Split9/1 -> pumpMotor_dataToIsr/Trigger
  tiltMotor_isrSchedule/1(Output) -> Function-Call Split11/1
  In Bus Element/1 -> allMotors_readAdc/1(PropMotorAdcFeedback)
  Function-Call Split5/1 -> pumpMotor_isrSchedule/Trigger
  Function-Call Split11/1 -> tiltMotor_dataToIsr/Trigger
  Function-Call Split7/1 -> tiltMotor_isrSchedule/Trigger
  Function-Call Split7/2 -> Function-Call Split5/1
  Function-Call Split14/2 -> Function-Call Split15/1
